simulink model "Lithium0x2Dion"  (R2024b)
settings: Solver=FixedStepAuto  StartTime=0.0  StopTime=1000  FixedStep=0.001  RelTol=1e-3
libraries: spsControlledCurrentSourceLib x1, spsControlledVoltageSourceLib x1, spsCurrentMeasurementLib x1, spsSeriesRLCBranchLib x1, spsVoltageMeasurementLib x1, sps_lib x1
(part 2 of 3)

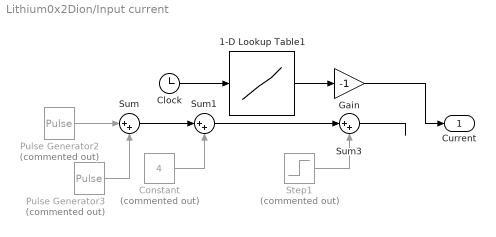
== system Lithium0x2Dion/Input current  ==
  1-D Lookup Table1 : Lookup_n-D  NumberOfTableDimensions=1  BreakpointsForDimension1=[0;1.01887913385872;2.0344900475502099;3.0500340296930499;4.0657185866475603;5.0810157495870998;6.0968101849684899;7.0968850778772303;8.1124882773801801;9.1126090294055793;10.1281133227785;11.143751965479201;12.1593450347718;13.1593660736653;14.1743463881394;15.1749018870141;16.1749419632797;17.190546205376499;18.1905584373526;19.190564844833698;20.190581668233801;21.205775288519401;22.221822783631101;23.2218732156689;24.237412155260198;25.2530114149558;26.268548790656499;27.2686751616639;28.2840278377444;29.284235480998198;30.299836620371899;31.299839002837;32.299865585522603;33.315439271584196;34.315444024949102;35.315493193840702;36.330888621312603;37.346691292186698;38.362012314501001;39.362300092165199;40.377961521564401;41.378030539854102;42.3935246428737;43.393526473970297;44.409117783881797;45.424770646965001;46.4400777496448;47.440356610113703;48.455970431045003;49.471618326770098;50.487212784515599;51.502824339811902;52.502837464009602;53.518261091652697;54.534072434107699;55.549677528320899;56.5652890535384;57.565310628768202;58.580888961390897;59.596420963716803;60.611908234732297;61.612151451510698;62.6277572374456;63.6433502165128;64.658985014644699;65.659028589616398;66.674502993610105;67.690219640422598;68.690297540811997;69.705869437420901;70.721430542165805;71.721433090046105;72.737097266286597;73.752713312755105;74.768296337049804;75.768298799714103;76.7838958138273;77.799575278106204;78.815131921754102;79.830762449259097;80.846361789153903;81.861982286704006;82.877665400064899;83.893241462032194;84.908964093738206;85.924478106295297;86.940101009830002;87.955695041517203;88.955702962768598;89.955753074013103;90.971291051206194;91.986979512876104;93.002588241131903;94.018159004914196;95.033664561437007;96.048809936659396;97.049413951266601;98.0650031709811;99.080407565765199;100.09631968399501;101.111465675753;102.11189873494;103.127516751312;104.143109544919;105.143124994898;106.158695713577;107.17431185528;108.18995113456501;109.189957511971;110.205781997138;111.221020358749;112.221212523484;113.221271506802;114.236735474828;115.252443846042;116.26771769096;117.26801012520799;118.268056487115;119.283640107897;120.29921178896301;121.299257875184;122.31477556189201;123.330453627696;124.346070576408;125.36168789604601;126.376858539144;127.37735104126099;128.39283488373999;129.39297683351501;130.408556048333;131.424146937199;132.439825594469;133.455381822085;134.45540407901001;135.47088355562701;136.47088728644999;137.486598690215;138.50225354826401;139.517838903361;140.533451170424;141.54906840485299;142.549084812221;143.56468928488499;144.58031647408299;145.59592787899999;146.59594247185299;147.61143503604401;148.62721970712701;149.642766050143;150.64278364546399;151.65835987785999;152.65836536305099;153.673986201444;154.68965248793;155.70525177269201;156.720359825038;157.72083801152601;158.73647469434599;159.75206754810301;160.752075288903;161.75209380150801;162.76767529198699;163.767718300551;164.78328856809799;165.798892389146;166.81450449581499;167.814555033114;168.82993256103899;169.84574065039899;170.84580755341801;171.86138725945801;172.877046177615;173.89259178880801;174.89260608090601;175.892665359967;176.908212159116;177.90821256666499;178.92379575136499;179.92381250960199;180.92383006482501;181.93940597140701;182.955051035086;183.955066129183;184.970642451804;185.97071898378999;186.98628896061601;188.00185918305201;189.01756192526199;190.03310776202099;191.048738800797;192.06438103743901;193.06441047222299;194.07997152183501;195.09552602515399;196.111195078534;197.11122443813301;198.12680355771201;199.12681930343001;200.14248037193801;201.15809403748099;202.15809915174401;203.173649239074;204.18907093190899;205.189275562658;206.20448673160701;207.20456485756199;208.20475768895301;209.220540635746;210.23609731448201;211.236120734298;212.25135854453799;213.26734386994599;214.26737208670201;215.267408142969;216.282924401115;217.28293268326499;218.29853800303999;219.31415405452199;220.31419412076499 ...(+193907 chars)]  Table=[0;-1.92431034520268e-05;-1.92431034520268e-05;-0.00019985238031949799;-1.92431034520268e-05;-1.92431034520268e-05;-1.92431034520268e-05;-1.92431034520268e-05;-1.92431034520268e-05;-1.92431034520268e-05;-1.92431034520268e-05;-1.92431034520268e-05;-1.92431034520268e-05;-1.92431034520268e-05;-1.92431034520268e-05;-1.92431034520268e-05;-1.92431034520268e-05;-0.49976509809494002;-0.49994572997093201;-0.49994572997093201;-0.49994572997093201;-0.49976509809494002;-0.49976509809494002;-0.49994572997093201;-0.50012630224227905;-0.49976509809494002;-0.49994572997093201;-0.49994572997093201;-0.49994572997093201;-0.49976509809494002;-0.49994572997093201;-0.49994572997093201;-0.49994572997093201;-0.49976509809494002;-0.49994572997093201;-0.49976509809494002;-0.49976509809494002;-0.49994572997093201;-0.49994572997093201;-0.49994572997093201;-0.49994572997093201;-0.49994572997093201;-0.49994572997093201;-0.50012630224227905;-0.49958449602127097;-1.00023341178894;-1.00023341178894;-1.0004140138626101;-1.00023341178894;-1.00023341178894;-1.0000528097152701;-1.00023341178894;-1.0000528097152701;-1.00023341178894;-1.0000528097152701;-1.00023341178894;-1.00023341178894;0.50026845932006803;0.50026845932006803;0.50044906139373802;0.50044906139373802;0.50026845932006803;0.50026845932006803;0.50026845932006803;0.50026845932006803;-1.92431034520268e-05;-1.92431034520268e-05;-1.92431034520268e-05;-1.92431034520268e-05;-1.92431034520268e-05;-1.92431034520268e-05;-1.92431034520268e-05;-1.92431034520268e-05;-1.92431034520268e-05;-1.92431034520268e-05;-1.92431034520268e-05;-1.92431034520268e-05;-1.92431034520268e-05;-1.92431034520268e-05;-1.92431034520268e-05;-1.92431034520268e-05;-0.49994572997093201;-0.49994572997093201;-0.49994572997093201;-0.49994572997093201;-0.50012630224227905;-0.49976509809494002;-0.49994572997093201;-0.49994572997093201;-0.49994572997093201;-0.50012630224227905;-0.49994572997093201;-0.49994572997093201;-0.49976509809494002;-0.49976509809494002;-0.49994572997093201;-0.49994572997093201;-0.49994572997093201;-0.49976509809494002;-0.49994572997093201;-0.49994572997093201;-0.50012630224227905;-0.49976509809494002;-0.49976509809494002;-0.49994572997093201;-0.49994572997093201;-0.49994572997093201;-0.49994572997093201;-0.49994572997093201;-0.49994572997093201;-0.49958449602127097;-0.50012630224227905;-0.49994572997093201;-0.49994572997093201;-0.49994572997093201;-0.49994572997093201;-0.49976509809494002;-0.49994572997093201;-0.49994572997093201;-0.49976509809494002;-0.49976509809494002;-0.50012630224227905;-0.49976509809494002;-0.49994572997093201;-0.49976509809494002;-0.49994572997093201;-0.49994572997093201;-0.49994572997093201;-0.49976509809494002;-0.49976509809494002;-0.49976509809494002;-0.49994572997093201;-0.49994572997093201;-0.49976509809494002;-0.49994572997093201;-0.49976509809494002;-0.49958449602127097;-0.49994572997093201;-0.49976509809494002;-0.49994572997093201;-0.49976509809494002;-0.49994572997093201;-0.49994572997093201;-0.49994572997093201;-0.49976509809494002;-0.49994572997093201;-0.49994572997093201;-0.50012630224227905;-0.49976509809494002;-0.49976509809494002;-0.49994572997093201;-0.49994572997093201;-0.49994572997093201;-0.49994572997093201;-0.49976509809494002;-0.49994572997093201;-0.49994572997093201;-0.49994572997093201;-0.49994572997093201;-0.49994572997093201;-0.49994572997093201;-0.49976509809494002;-0.49994572997093201;-0.49994572997093201;-0.49994572997093201;-0.49994572997093201;-0.49994572997093201;-0.49976509809494002;-1.00023341178894;-1.0000528097152701;-1.00023341178894;-1.0004140138626101;-1.00023341178894;-0.99987220764160201;-1.0000528097152701;-1.00023341178894;-1.00023341178894;-1.00023341178894;-1.0000528097152701;-1.00023341178894;0.50026845932006803;0.50026845932006803;0.50026845932006803;0.50008785724639904;0.50026845932006803;0.50008785724639904;0.50044906139373802;0.50026845932006803;-1.92431034520268e-05;-1.92431034520268e-05;-1.92431034520268e-05;-1.92431034520268e-05 ...(+216021 chars)]  InternalRulePriority=Speed  RndMeth=Simplest
  Clock : Clock
  Constant : Constant  Commented=on  Value=4
  Gain : Gain  Gain=-1
  Pulse Generator2 : DiscretePulseGenerator  Commented=on  PulseType=Time based  Amplitude=2.35  Period=3600  PulseWidth=50
  Pulse Generator3 : DiscretePulseGenerator  Commented=on  PulseType=Time based  Amplitude=-4.7  Period=3600  PulseWidth=50  PhaseDelay=3600
  Step1 : Step  Commented=on  Time=1800  After=-8  SampleTime=0
  Sum : Sum  Inputs=|++
  Sum1 : Sum  Inputs=|++
  Sum3 : Sum  Inputs=|++
  Current : Outport
  wires:
  Constant/1 -> Sum1/2
  Step1/1 -> Sum3/2
  Sum3/1 -> ?
  Pulse Generator2/1 -> Sum/1
  Sum/1 -> Sum1/1
  Pulse Generator3/1 -> Sum/2
  Sum1/1 -> Sum3/1
  1-D Lookup Table1/1 -> Gain/1
  Clock/1 -> 1-D Lookup Table1/1
  Gain/1 -> Current/1
